simulink model "sk_R3GDL"  (Simulink 9.0)
settings: Solver=ode45  StartTime=0.0  StopTime=10  MaxStep=1e-3  RelTol=1e-3  EnableMultiTasking=on
settings Model: Creator=mortega  LastModifiedBy=fevaf  ExtModeTrigMode=oneshot  ExtModeArmWhenConnect=off
settings DataIOCC: SignalLoggingSaveFormat=ModelDataLogs
settings OptimizationCC: BlockReduction=off  BooleanDataType=off  ExpressionDepthLimit=2147483647  InitFltsAndDblsToZero=on
settings DebuggingCC: SaveWithParameterizedLinksMsg=none  SignalResolutionControl=TryResolveAllWithWarning  MultiTaskDSMMsg=warning  MultiTaskCondExecSysMsg=none  FcnCallInpInsideContextMsg=warning  StateNameClashWarn=warning  StrictBusMsg=None
settings HardwareCC: TargetUnknown=on
settings GRTTargetCC: TargetFcnLib=ansi_tfl_tmw.mat  CombineOutputUpdateFcns=off  GRTInterface=on

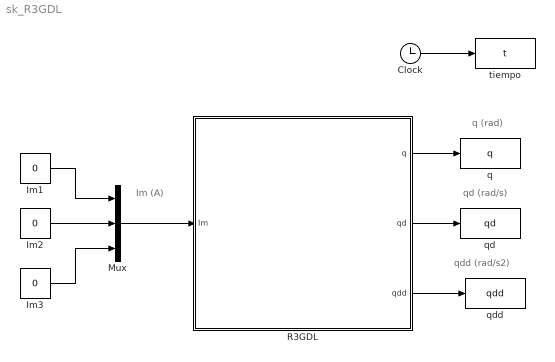
== system sk_R3GDL ==
  note: Im (A)
  note: q (rad)
  note: qd (rad/s)
  note: qdd (rad/s2)
  Clock : Clock
  Im1 : Constant  Value=0
  Im2 : Constant  Value=0
  Im3 : Constant  Value=0
  Mux : Mux  Inputs=3
  R3GDL : Subsystem  mask(Control y Programación de Robots (4 GIERM)){NGrupo=3, q1_ini=0, q2_ini=0, q3_ini=0, Bl_q1=off, Bl_q2=off, Bl_q3=off, AccionamientoDirecto=off}
      mask prompts: NGrupo "Nº de GRUPO"; q1_ini "q1 inicial  (rad)"; q2_ini "q2 inicial (rad)"; q3_ini "q3_inicial (rad)"; Bl_q1 "Bloqueo q1"; Bl_q2 "Bloqueo q2"; Bl_q3 "Bloqueo q3"; AccionamientoDirecto "Accionamiento directo"
      mask help: Robot de 3 grados de libertad RRR
      mask Display:
      | image(imread('R3GDL_RRR.JPG'));
      | port_label('output', 1, 'q');
      | port_label('output', 2, 'qd');
      | port_label('output', 3, 'qdd');
      | port_label('input', 1, 'Im')
  q : ToWorkspace  VariableName=q  SampleTime=-1
  qd : ToWorkspace  VariableName=qd  SampleTime=-1
  qdd : ToWorkspace  VariableName=qdd  SampleTime=-1
  tiempo : ToWorkspace  VariableName=t  SampleTime=-1
  wires:
  Clock/1 -> tiempo/1
  Mux/1 -> R3GDL/1(Im)
  R3GDL/1(q) -> q/1
  R3GDL/2(qd) -> qd/1
  R3GDL/3(qdd) -> qdd/1
  Im2/1 -> Mux/2
  Im1/1 -> Mux/1
  Im3/1 -> Mux/3

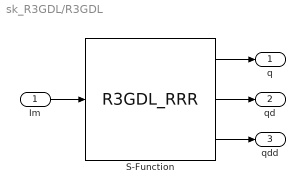
== system sk_R3GDL/R3GDL ==
  Im : Inport
  S-Function : S-Function  FunctionName=R3GDL_RRR  Parameters=[q1_ini; q2_ini; q3_ini]; [Bl_q1; Bl_q2; Bl_q3]; AccionamientoDirecto; NGrupo  SFunctionDeploymentMode=off  EnableBusSupport=off
  q : Outport
  qd : Outport  Port=2
  qdd : Outport  Port=3
  wires:
  Im/1 -> S-Function/1
  S-Function/1 -> q/1
  S-Function/2 -> qd/1
  S-Function/3 -> qdd/1
